simulink model "for_demo"  (R2014a)
settings: Solver=FixedStepDiscrete  StartTime=0.0  StopTime=10.0  FixedStep=0.1  RelTol=1e-3
settings Model: Creator=yoshi12  LastModifiedBy=yoshi12

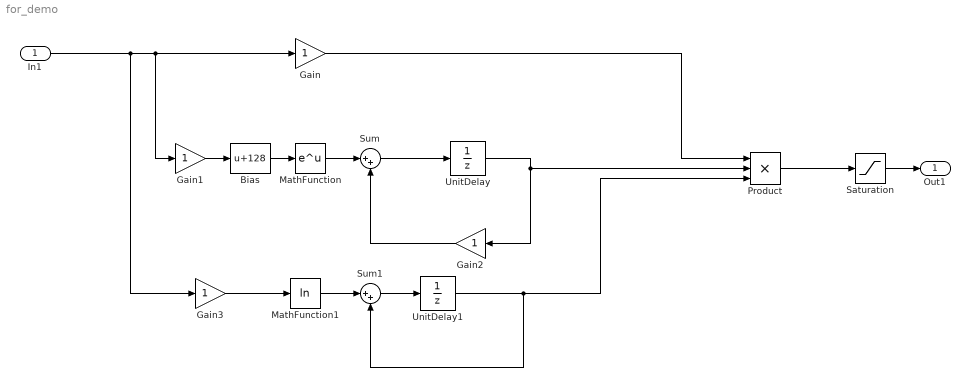
== system for_demo ==
  In1 : Inport
  Bias : Bias  Bias=128
  Gain{,1..3} (4 alike) : Gain
  MathFunction : Math  SaturateOnIntegerOverflow=on
  MathFunction1 : Math  Operator=log  SaturateOnIntegerOverflow=on
  Product : Product  Inputs=3
  Saturation : Saturate
  Sum : Sum  Inputs=|++
  Sum1 : Sum  Inputs=|++
  UnitDelay : UnitDelay  SampleTime=-1
  UnitDelay1 : UnitDelay  SampleTime=-1
  Out1 : Outport
  wires:
  In1/1 -> Gain1/1, Gain/1, Gain3/1
  Gain/1 -> Product/1
  Product/1 -> Saturation/1
  Saturation/1 -> Out1/1
  Gain1/1 -> Bias/1
  Gain3/1 -> MathFunction1/1
  MathFunction1/1 -> Sum1/1
  UnitDelay1/1 -> Sum1/2, Product/3
  Sum1/1 -> UnitDelay1/1
  UnitDelay/1 -> Gain2/1, Product/2
  MathFunction/1 -> Sum/1
  Gain2/1 -> Sum/2
  Bias/1 -> MathFunction/1
  Sum/1 -> UnitDelay/1
